simulink model "Invertibilidad"  (R2023b)
settings: Solver=VariableStepAuto  StartTime=0.0  StopTime=4  RelTol=1e-3
settings Model: Creator=Alejandro Villeda  LastModifiedBy=Alejandro Villeda

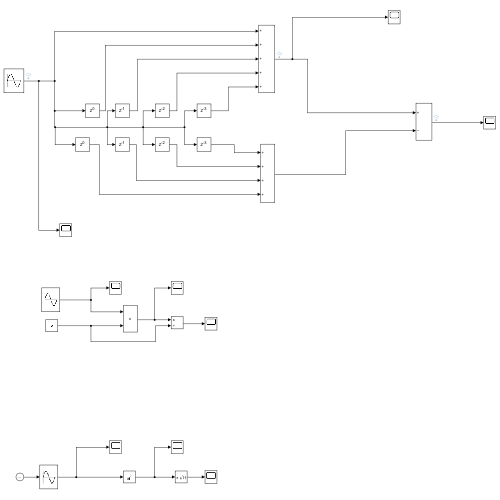
[thumbnail: Simulink's stored preview of the top-level diagram]
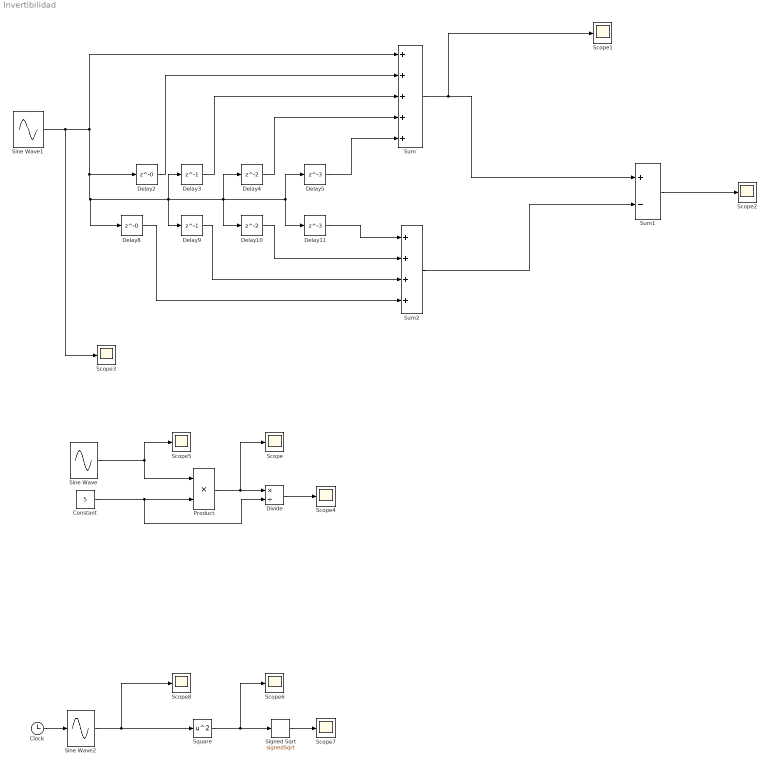
== system Invertibilidad ==
  Clock : Clock
  Constant : Constant  Value=5
  Delay10 : Delay  InitialCondition=0
  Delay11 : Delay  DelayLength=3  InitialCondition=0
  Delay2 : Delay  DelayLength=0  InitialCondition=0
  Delay3 : Delay  DelayLength=1  InitialCondition=0
  Delay4 : Delay  InitialCondition=0
  Delay5 : Delay  DelayLength=3  InitialCondition=0
  Delay8 : Delay  DelayLength=0  InitialCondition=0
  Delay9 : Delay  DelayLength=1  InitialCondition=0
  Divide : Product  Inputs=*/
  Product : Product
  Scope{,1..8} (9 alike) : Scope
  Signed Sqrt : Sqrt  Operator=signedSqrt  OutputSignalType=real  RndMeth=Nearest
  Sine Wave : Sin  Frequency=pi  SampleTime=0
  Sine Wave1 : Sin  Frequency=pi  SampleTime=0
  Sine Wave2 : Sin  TimeSource=Use external signal  Frequency=pi  SampleTime=0
  Square : Math  Operator=square
  Sum : Sum  Inputs=+++++
  Sum1 : Sum  Inputs=+-
  Sum2 : Sum  Inputs=++++
  wires:
  Delay2/1 -> Sum/2
  Delay3/1 -> Sum/3
  Delay4/1 -> Sum/4
  Delay5/1 -> Sum/5
  Sum/1 -> Sum1/1, Scope1/1
  Sum1/1 -> Scope2/1
  Sine Wave1/1 -> Scope3/1, Delay8/1, Delay9/1, Delay3/1, Delay10/1, Delay4/1, Delay11/1, Delay5/1, Delay2/1, Sum/1
  Delay11/1 -> Sum2/1
  Delay10/1 -> Sum2/2
  Delay9/1 -> Sum2/3
  Delay8/1 -> Sum2/4
  Sum2/1 -> Sum1/2
  Product/1 -> Scope/1, Divide/1
  Sine Wave/1 -> Product/1, Scope5/1
  Constant/1 -> Divide/2, Product/2
  Divide/1 -> Scope4/1
  Sine Wave2/1 -> Square/1, Scope8/1
  Signed Sqrt/1 -> Scope7/1
  Square/1 -> Signed Sqrt/1, Scope6/1
  Clock/1 -> Sine Wave2/1
